simulink model "questao3MiguelThamiresPaiva"  (Simulink 8.1)
settings: Solver=ode45  StartTime=0.0  StopTime=20  MaxStep=0.01  RelTol=1e-3
values from neighbouring files (symbols this model uses):
  A = [0 1  0              0 ... (first row only)    [MatLab4p.m]    (also in MatLab5p.m = [     0        1       0        0; MatLab6p_solucao4.m = [     0        1       0        0; MatLab7p.m = [0 1; -5*sqrt(2) -1]; pplane8.m = [)
  Am = blkdiag(M,M)    [MatLab5p.m]    (also in MatLab6p_solucao4.m; questao2Miguel.m = blkdiag(M); questao2MiguelFinal.m = blkdiag(M))
  B = [0; 1/M; 0; -1/(M*L)]    [MatLab4p.m]    (also in MatLab5p.m = [ 0    0; MatLab6p_solucao4.m = [ 0    0; MatLab7p.m = [0 ; 10]; pplane8.m = real(A))
  Bm = blkdiag(N,N)    [MatLab5p.m]    (also in MatLab6p_solucao4.m; questao2Miguel.m = blkdiag(N); questao2MiguelFinal.m = blkdiag(N))
  C = [1 0 0 0]    [MatLab4p.m]    (also in MatLab5p.m = [1 0 0 0; MatLab6p_solucao4.m = [1 0 0 0; MatLab7p.m = [1 0]; pplane8.m = imag(A))
  g = 9.81    [MatLab4p.m]    (also in PenduloInvertidoNLinear.m; questao2Miguel.m; questao2MiguelFinal.m)
  K = place(A,B,[-3 -3.05 -3.1 -3.15])    [MatLab4p.m]    (also in MatLab5p.m = Ka(:,1:4); MatLab6p_solucao4.m = Ka(:,1:4); MatLab7p.m = place(A,B,[-4 -4.05]); pplane8.m = kk +2*(jj-1))
  Km = Ka(:,5:10)    [MatLab5p.m]    (also in MatLab6p_solucao4.m = Ka(:,5:12); MatLab7p.m = Ka(1,3); questao2Miguel.m = Ka(5); questao2MiguelFinal.m = Ka(5))
  L = (place(A',C',[-9 -9.05 -9.1 -9.15]))'    [MatLab4p.m]    (also in MatLab7p.m = [23 ; 113.9289]; PenduloInvertidoNLinear.m = 1; pplane8.m = length(t); questao2Miguel.m = 1)
  Lobs = H'    [MatLab6p_solucao4.m]    (also in questao2Miguel.m; questao2MiguelFinal.m)
  m = 0.5    [MatLab4p.m]    (also in PenduloInvertidoNLinear.m; questao2Miguel.m; questao2MiguelFinal.m)
  Mcar = 1    [questao2MiguelFinal.m]
  x0 = [0 0 pi/4 0]    [MatLab4p.m]    (also in MatLab5p.m = [1 0.5 1 0.1]; MatLab6p_solucao4.m = [0 0 0 0]; MatLab7p.m = [0 ; 0]; questao2Miguel.m = [0 0.01 0.3 0])
  x0obs = [0 0 0 0]    [MatLab4p.m]    (also in MatLab6p_solucao4.m; MatLab7p.m = [0 ; 0]; questao2Miguel.m; questao2MiguelFinal.m)
settings Model: Creator=hector  LastModifiedBy=Deinis-UFSC
settings DataIOCC: SignalLoggingSaveFormat=Dataset
settings OptimizationCC: ExpressionDepthLimit=128
settings DebuggingCC: UnderspecifiedInitializationDetection=Simplified  MergeDetectMultiDrivingBlocksExec=error  FcnCallInpInsideContextMsg=EnableAllAsError  FrameProcessingCompatibilityMsg=error  StateNameClashWarn=none
settings GRTTargetCC: CodeReplacementLibrary=C89/C90 (ANSI)  CombineOutputUpdateFcns=on  GRTInterface=off

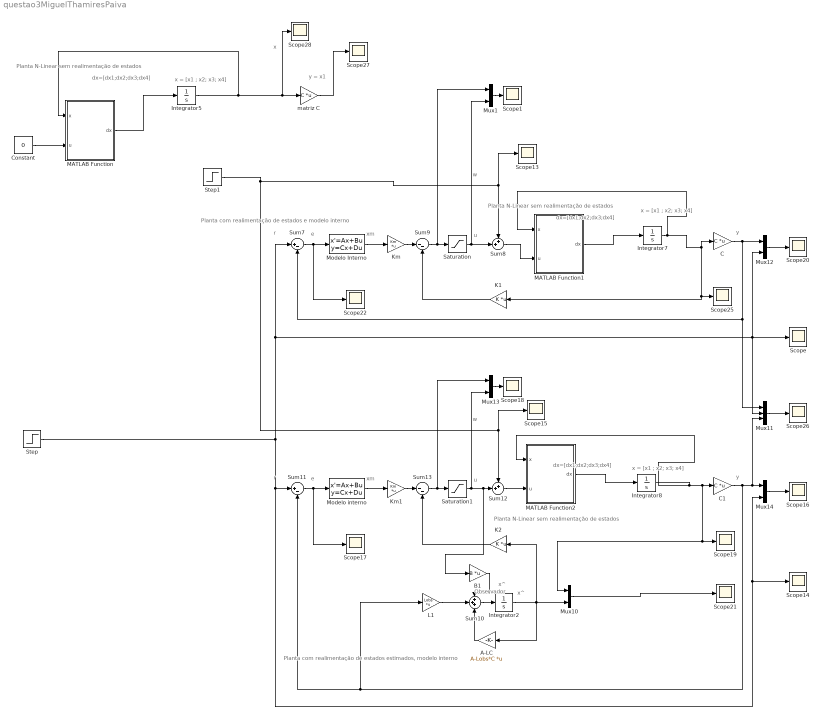
== system questao3MiguelThamiresPaiva ==
  note: Planta com realimentação de estados estimados, modelo interno
  note: Planta com realimentação de estados e modelo interno
  note: w
  note: u
  note: xm
  note: e
  note: r
  note: y
  note: w
  note: u
  note: xm
  note: e
  note: r
  note: y
  note: Observador
  note: x^
  note: x^
  note: Planta N-Linear sem realimentação de estados
  note: x
  note: y = x1
  note: dx=[dx1;dx2;dx3;dx4]
  note: x = [x1 ; x2; x3; x4]
  note: Planta N-Linear sem realimentação de estados
  note: dx=[dx1;dx2;dx3;dx4]
  note: x = [x1 ; x2; x3; x4]
  note: Planta N-Linear sem realimentação de estados
  note: dx=[dx1;dx2;dx3;dx4]
  note: x = [x1 ; x2; x3; x4]
  A-LC : Gain  Gain=A-Lobs*C  Multiplication=Matrix(K*u)
  B1 : Gain  Gain=B  Multiplication=Matrix(K*u)
  C : Gain  Gain=C  Multiplication=Matrix(K*u)
  C1 : Gain  Gain=C  Multiplication=Matrix(K*u)
  Constant : Constant  Value=0
  Integrator2 : Integrator  InitialCondition=x0obs
  Integrator5 : Integrator  InitialCondition=x0
  Integrator7 : Integrator  InitialCondition=x0
  Integrator8 : Integrator  InitialCondition=[0;0;0.01;0]
  K1 : Gain  Gain=K  Multiplication=Matrix(K*u)
  K2 : Gain  Gain=K  Multiplication=Matrix(K*u)
  Km : Gain  Gain=Km  Multiplication=Matrix(K*u)
  Km1 : Gain  Gain=Km  Multiplication=Matrix(K*u)
  L1 : Gain  Gain=Lobs  Multiplication=Matrix(K*u)
  MATLAB Function : MATLAB Function  TreatAsAtomicUnit=on
      settings: PermitHierarchicalResolution=ParametersOnly
  MATLAB Function1 : MATLAB Function  TreatAsAtomicUnit=on
      settings: PermitHierarchicalResolution=ParametersOnly
  MATLAB Function2 : MATLAB Function  TreatAsAtomicUnit=on
      settings: PermitHierarchicalResolution=ParametersOnly
  Modelo Interno : StateSpace  A=Am  B=Bm  D=0  X0=0
  Modelo interno : StateSpace  A=Am  B=Bm  D=0  X0=0
  Mux{1,10,12..14} (5 alike) : Mux  Inputs=2
  Mux11 : Mux  Inputs=3
  Saturation : Saturate  UpperLimit=50  LowerLimit=-50
  Saturation1 : Saturate  UpperLimit=50  LowerLimit=-50
  Scope{,1,13..22,25..28} (16 alike) : Scope
      Scope settings: TimeRange=auto  MaxDataPoints=5000  SaveToWorkspace=off  SaveName=ScopeData14  YMin=-10  YMax=10  SampleTime=-1  DataFormat=Array
      Scope1 settings: TimeRange=auto  MaxDataPoints=5000  SaveToWorkspace=off  SaveName=ScopeData  YMin=-41.9288  YMax=84.74678  SampleTime=-1  DataFormat=Array
      Scope13 settings: TimeRange=auto  MaxDataPoints=5000  SaveToWorkspace=off  SaveName=ScopeData15  YMin=-10  YMax=10  SampleTime=-1  DataFormat=Array
      Scope14 settings: TimeRange=auto  MaxDataPoints=5000  SaveToWorkspace=off  SaveName=ScopeData16  YMin=-10  YMax=10  SampleTime=-1  DataFormat=Array
      Scope15 settings: TimeRange=auto  MaxDataPoints=5000  SaveToWorkspace=off  SaveName=ScopeData17  YMin=-10  YMax=10  SampleTime=-1  DataFormat=Array
      Scope16 settings: TimeRange=auto  MaxDataPoints=5000  SaveToWorkspace=off  SaveName=ScopeData18  YMin=-7155.17691  YMax=798.36109  SampleTime=-1  DataFormat=Array
      Scope17 settings: TimeRange=auto  MaxDataPoints=5000  SaveToWorkspace=off  SaveName=ScopeData19  YMin=-10  YMax=10  SampleTime=-1
      Scope18 settings: TimeRange=auto  MaxDataPoints=5000  SaveToWorkspace=off  SaveName=ScopeData20  YMin=-40789.71039  YMax=38956.08741  SampleTime=-1  DataFormat=Array
      Scope19 settings: TimeRange=auto  ShowLegends=on  LimitDataPoints=on  MaxDataPoints=5000  SaveToWorkspace=off  SaveName=ScopeData21  YMin=-7.81953  YMax=14.72912  SampleTime=-1
      Scope20 settings: TimeRange=auto  MaxDataPoints=5000  SaveToWorkspace=off  SaveName=ScopeData22  YMin=-0.46447  YMax=1.16445  SampleTime=-1
      Scope21 settings: TimeRange=auto  MaxDataPoints=5000  SaveToWorkspace=off  SaveName=ScopeData23  YMin=-90.00724  YMax=72.94729  SampleTime=-1
      Scope22 settings: TimeRange=auto  MaxDataPoints=5000  SaveToWorkspace=off  SaveName=ScopeData24  YMin=-10  YMax=10  SampleTime=-1
      Scope25 settings: TimeRange=auto  ShowLegends=on  LimitDataPoints=on  MaxDataPoints=5000  SaveToWorkspace=off  SaveName=ScopeData27  YMin=-0.5  YMax=3.25  SampleTime=-1
      Scope26 settings: TimeRange=auto  ShowLegends=on  MaxDataPoints=5000  SaveToWorkspace=off  SaveName=ScopeData28  YMin=-0.54659  YMax=1.90348  SampleTime=-1  DataFormat=Array
      Scope27 settings: TimeRange=auto  MaxDataPoints=5000  SaveToWorkspace=off  SaveName=ScopeData29  YMin=4.00000  YMax=6.00000  SampleTime=-1
      Scope28 settings: TimeRange=auto  MaxDataPoints=5000  SaveToWorkspace=off  SaveName=ScopeData30  YMin=-9.4823  YMax=9.48205  SampleTime=-1
  Step : Step  Time=5  SampleTime=0
  Step1 : Step  Time=15  After=0.3  SampleTime=0
  Sum10 : Sum  Inputs=+++
  Sum11 : Sum  Inputs=|+-
  Sum12 : Sum  Inputs=++|
  Sum13 : Sum  Inputs=|--
  Sum7 : Sum  Inputs=|+-
  Sum8 : Sum  Inputs=++|
  Sum9 : Sum  Inputs=|--
  matriz C : Gain  Gain=C  Multiplication=Matrix(K*u)
  wires:
  Sum7/1 -> Modelo Interno/1, Scope22/1
  Mux12/1 -> Scope20/1
  Km/1 -> Sum9/1
  Modelo Interno/1 -> Km/1
  K1/1 -> Sum9/2
  Step/1 -> Sum7/1, Mux11/2, Scope/1, Mux12/2, Sum11/1, Scope14/1, Mux14/2
  Sum11/1 -> Modelo interno/1, Scope17/1
  Step1/1 -> Sum12/1, Scope15/1, Sum8/1, Scope13/1
  Mux14/1 -> Scope16/1
  Sum13/1 -> Mux13/1, Saturation1/1
  Km1/1 -> Sum13/1
  Modelo interno/1 -> Km1/1
  K2/1 -> Sum13/2
  Sum10/1 -> Integrator2/1
  L1/1 -> Sum10/2
  A-LC/1 -> Sum10/3
  B1/1 -> Sum10/1
  Mux10/1 -> Scope21/1
  Mux11/1 -> Scope26/1
  matriz C/1 -> Scope27/1
  Mux13/1 -> Scope18/1
  Constant/1 -> MATLAB Function/2(u)
  Sum8/1 -> MATLAB Function1/2(u)
  MATLAB Function1/1(dx) -> Integrator7/1
  Sum12/1 -> MATLAB Function2/2(u)
  MATLAB Function2/1(dx) -> Integrator8/1
  C1/1 -> L1/1, Sum11/2, Mux11/3, Mux14/1
  C/1 -> Mux12/1, Sum7/2, Mux11/1
  Integrator5/1 -> MATLAB Function/1(x), Scope28/1, matriz C/1
  Integrator7/1 -> MATLAB Function1/1(x), K1/1, Scope25/1, C/1
  Saturation1/1 -> Mux13/2, B1/1, Sum12/2
  Integrator2/1 -> A-LC/1, Mux10/2, K2/1
  Integrator8/1 -> Mux10/1, Scope19/1, C1/1, MATLAB Function2/1(x)
  MATLAB Function/1(dx) -> Integrator5/1
  Sum9/1 -> Mux1/1, Saturation/1
  Mux1/1 -> Scope1/1
  Saturation/1 -> Mux1/2, Sum8/2

== matlab function MATLAB Function1 ==
  data: x input double; u input double; dx output double; m parameter double; Mcar parameter double; L parameter double; g parameter double
function dx = fcn(x,u,m, Mcar, L, g)
%#codegen

dx1 = x(2);
dx2 = u - (m*g*cos(x(3))*sin(x(3))+m*L*x(4)^2*sin(x(3)))/(Mcar+m - m*cos(x(3))^2);
dx3 = x(4);
dx4 = (u*cos(x(3))+m*L*x(4)^2*cos(x(3))*sin(x(3))-(Mcar+m)*g*sin(x(3)))/(m*L*cos(x(3))^2 - L*(Mcar+m));

dx = [dx1 ; dx2 ; dx3 ; dx4];

== matlab function MATLAB Function ==
  data: x input double; u input double; dx output double; m parameter double; Mcar parameter double; L parameter double; g parameter double
function dx = fcn(x,u,m, Mcar, L, g)
%#codegen

dx1 = x(2);
dx2 = u - (m*g*cos(x(3))*sin(x(3))+m*L*x(4)^2*sin(x(3)))/(Mcar+m - m*cos(x(3))^2);
dx3 = x(4);
dx4 = (u*cos(x(3))+m*L*x(4)^2*cos(x(3))*sin(x(3))-(Mcar+m)*g*sin(x(3)))/(m*L*cos(x(3))^2 - L*(Mcar+m));

dx = [dx1 ; dx2 ; dx3 ; dx4];

== matlab function MATLAB Function2 ==
  data: x input double; u input double; dx output double; m parameter double; Mcar parameter double; L parameter double; g parameter double
function dx = fcn(x,u,m, Mcar, L, g)
%#codegen

dx1 = x(2);
dx2 = u - (m*g*cos(x(3))*sin(x(3))+m*L*x(4)^2*sin(x(3)))/(Mcar+m - m*cos(x(3))^2);
dx3 = x(4);
dx4 = (u*cos(x(3))+m*L*x(4)^2*cos(x(3))*sin(x(3))-(Mcar+m)*g*sin(x(3)))/(m*L*cos(x(3))^2 - L*(Mcar+m));

dx = [dx1 ; dx2 ; dx3 ; dx4];
